simulink model "nlm_1"  (Simulink 5.0)
settings: Solver=ode45  StartTime=0.0  StopTime=600  RelTol=1e-3
libraries: dspsigops x17, fixpt_lib_4 x4
settings Model: Creator=svenhoffmann  LastModifiedBy=svenhoffmann  ExtModeAutoUpdateStatusClock=off  OutputSaveName=yp

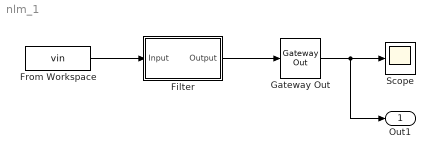
== system nlm_1 ==
  Filter : Subsystem  Tag=FilterWizardSubSystem
  From Workspace : FromWorkspace  VariableName=vin  SampleTime=1
  Gateway Out : fixpt_lib_4/Data Type/Gateway Out  OutRealWorld=Real World Value  OutBuiltInType=double  DoSatur=off
  Scope : Scope
      settings: TimeRange=600  YMin=-0.1  YMax=0.15
  Out1 : Outport
  wires:
  From Workspace/1 -> Filter/1(Input)
  Filter/1(Output) -> Gateway Out/1
  Gateway Out/1 -> Scope/1, Out1/1

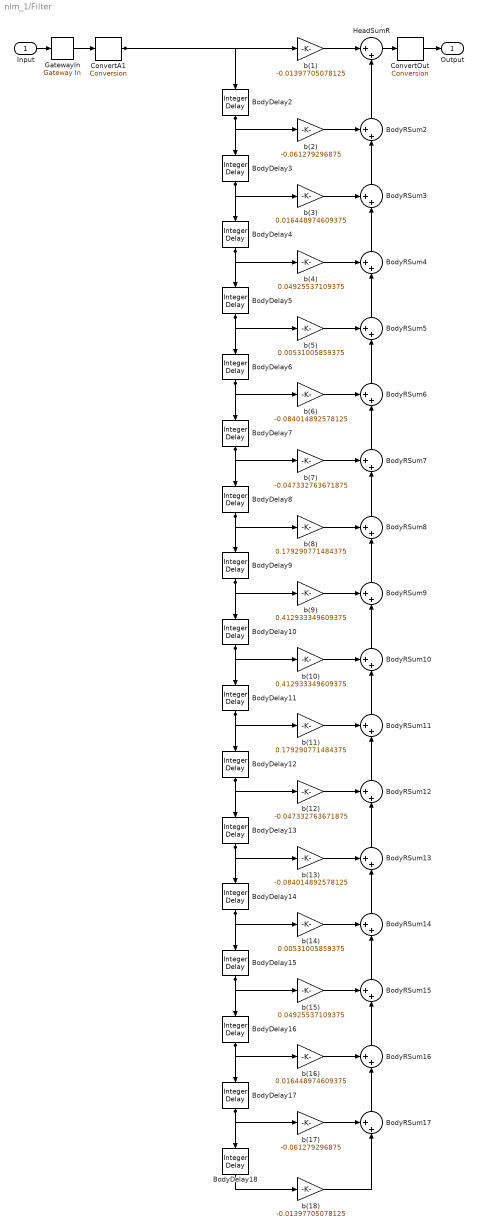
== system nlm_1/Filter ==
  Input : Inport
  BodyDelay{2..18} (17 alike) : dspsigops/Integer Delay  Orientation=down  delay=1  ic=0  reset_popup=None
  BodyRSum{2..17} (16 alike) : Sum  Orientation=up  Inputs=++|  ShowAdditionalParam=on  OutDataTypeMode=Specify via dialog  OutDataType=sfix(32)  OutScaling=2^-30  SaturateOnIntegerOverflow=on  LockScale=on
  ConvertA1 : fixpt_lib_4/Data Type/Conversion  ConvertRealWorld=Real World Value  OutputDataTypeScalingMode=Specify via dialog  OutDataType=sfix(16)  OutScaling=2^-15  DoSatur=on
      settings: LockScale=on
  ConvertOut : fixpt_lib_4/Data Type/Conversion  ConvertRealWorld=Real World Value  OutputDataTypeScalingMode=Specify via dialog  OutDataType=sfix(16)  OutScaling=2^-15  DoSatur=on
      settings: LockScale=on
  GatewayIn : fixpt_lib_4/Data Type/Gateway In  InRealWorld=Real World Value  OutputDataTypeScalingMode=Specify via dialog  OutDataType=sfix(16)  OutScaling=2^-15  DoSatur=on
      settings: LockScale=on
  HeadSumR : Sum  Inputs=|++  ShowAdditionalParam=on  OutDataTypeMode=Specify via dialog  OutDataType=sfix(32)  OutScaling=2^-30  SaturateOnIntegerOverflow=on  LockScale=on
  b(1) : Gain  Gain=-0.01397705078125  ShowAdditionalParam=on  ParameterDataType=float('double')  OutDataTypeMode=Specify via dialog  OutScaling=2^-15  SaturateOnIntegerOverflow=on  LockScale=on
  b(10) : Gain  Gain=0.412933349609375  ShowAdditionalParam=on  ParameterDataType=float('double')  OutDataTypeMode=Specify via dialog  OutScaling=2^-15  SaturateOnIntegerOverflow=on  LockScale=on
  b(11) : Gain  Gain=0.179290771484375  ShowAdditionalParam=on  ParameterDataType=float('double')  OutDataTypeMode=Specify via dialog  OutScaling=2^-15  SaturateOnIntegerOverflow=on  LockScale=on
  b(12) : Gain  Gain=-0.047332763671875  ShowAdditionalParam=on  ParameterDataType=float('double')  OutDataTypeMode=Specify via dialog  OutScaling=2^-15  SaturateOnIntegerOverflow=on  LockScale=on
  b(13) : Gain  Gain=-0.084014892578125  ShowAdditionalParam=on  ParameterDataType=float('double')  OutDataTypeMode=Specify via dialog  OutScaling=2^-15  SaturateOnIntegerOverflow=on  LockScale=on
  b(14) : Gain  Gain=0.00531005859375  ShowAdditionalParam=on  ParameterDataType=float('double')  OutDataTypeMode=Specify via dialog  OutScaling=2^-15  SaturateOnIntegerOverflow=on  LockScale=on
  b(15) : Gain  Gain=0.04925537109375  ShowAdditionalParam=on  ParameterDataType=float('double')  OutDataTypeMode=Specify via dialog  OutScaling=2^-15  SaturateOnIntegerOverflow=on  LockScale=on
  b(16) : Gain  Gain=0.016448974609375  ShowAdditionalParam=on  ParameterDataType=float('double')  OutDataTypeMode=Specify via dialog  OutScaling=2^-15  SaturateOnIntegerOverflow=on  LockScale=on
  b(17) : Gain  Gain=-0.061279296875  ShowAdditionalParam=on  ParameterDataType=float('double')  OutDataTypeMode=Specify via dialog  OutScaling=2^-15  SaturateOnIntegerOverflow=on  LockScale=on
  b(18) : Gain  Gain=-0.01397705078125  ShowAdditionalParam=on  ParameterDataType=float('double')  OutDataTypeMode=Specify via dialog  OutScaling=2^-15  SaturateOnIntegerOverflow=on  LockScale=on
  b(2) : Gain  Gain=-0.061279296875  ShowAdditionalParam=on  ParameterDataType=float('double')  OutDataTypeMode=Specify via dialog  OutScaling=2^-15  SaturateOnIntegerOverflow=on  LockScale=on
  b(3) : Gain  Gain=0.016448974609375  ShowAdditionalParam=on  ParameterDataType=float('double')  OutDataTypeMode=Specify via dialog  OutScaling=2^-15  SaturateOnIntegerOverflow=on  LockScale=on
  b(4) : Gain  Gain=0.04925537109375  ShowAdditionalParam=on  ParameterDataType=float('double')  OutDataTypeMode=Specify via dialog  OutScaling=2^-15  SaturateOnIntegerOverflow=on  LockScale=on
  b(5) : Gain  Gain=0.00531005859375  ShowAdditionalParam=on  ParameterDataType=float('double')  OutDataTypeMode=Specify via dialog  OutScaling=2^-15  SaturateOnIntegerOverflow=on  LockScale=on
  b(6) : Gain  Gain=-0.084014892578125  ShowAdditionalParam=on  ParameterDataType=float('double')  OutDataTypeMode=Specify via dialog  OutScaling=2^-15  SaturateOnIntegerOverflow=on  LockScale=on
  b(7) : Gain  Gain=-0.047332763671875  ShowAdditionalParam=on  ParameterDataType=float('double')  OutDataTypeMode=Specify via dialog  OutScaling=2^-15  SaturateOnIntegerOverflow=on  LockScale=on
  b(8) : Gain  Gain=0.179290771484375  ShowAdditionalParam=on  ParameterDataType=float('double')  OutDataTypeMode=Specify via dialog  OutScaling=2^-15  SaturateOnIntegerOverflow=on  LockScale=on
  b(9) : Gain  Gain=0.412933349609375  ShowAdditionalParam=on  ParameterDataType=float('double')  OutDataTypeMode=Specify via dialog  OutScaling=2^-15  SaturateOnIntegerOverflow=on  LockScale=on
  Output : Outport
  wires:
  GatewayIn/1 -> ConvertA1/1
  Input/1 -> GatewayIn/1
  ConvertOut/1 -> Output/1
  HeadSumR/1 -> ConvertOut/1
  ConvertA1/1 -> b(1)/1, BodyDelay2/1
  b(18)/1 -> BodyRSum17/2
  BodyDelay18/1 -> b(18)/1
  BodyRSum17/1 -> BodyRSum16/2
  b(17)/1 -> BodyRSum17/1
  BodyDelay17/1 -> BodyDelay18/1, b(17)/1
  BodyRSum16/1 -> BodyRSum15/2
  b(16)/1 -> BodyRSum16/1
  BodyDelay16/1 -> BodyDelay17/1, b(16)/1
  BodyRSum15/1 -> BodyRSum14/2
  b(15)/1 -> BodyRSum15/1
  BodyDelay15/1 -> BodyDelay16/1, b(15)/1
  BodyRSum14/1 -> BodyRSum13/2
  b(14)/1 -> BodyRSum14/1
  BodyDelay14/1 -> BodyDelay15/1, b(14)/1
  BodyRSum13/1 -> BodyRSum12/2
  b(13)/1 -> BodyRSum13/1
  BodyDelay13/1 -> BodyDelay14/1, b(13)/1
  BodyRSum12/1 -> BodyRSum11/2
  b(12)/1 -> BodyRSum12/1
  BodyDelay12/1 -> BodyDelay13/1, b(12)/1
  BodyRSum11/1 -> BodyRSum10/2
  b(11)/1 -> BodyRSum11/1
  BodyDelay11/1 -> BodyDelay12/1, b(11)/1
  BodyRSum10/1 -> BodyRSum9/2
  b(10)/1 -> BodyRSum10/1
  BodyDelay10/1 -> BodyDelay11/1, b(10)/1
  BodyRSum9/1 -> BodyRSum8/2
  b(9)/1 -> BodyRSum9/1
  BodyDelay9/1 -> BodyDelay10/1, b(9)/1
  BodyRSum8/1 -> BodyRSum7/2
  b(8)/1 -> BodyRSum8/1
  BodyDelay8/1 -> BodyDelay9/1, b(8)/1
  BodyRSum7/1 -> BodyRSum6/2
  b(7)/1 -> BodyRSum7/1
  BodyDelay7/1 -> BodyDelay8/1, b(7)/1
  BodyRSum6/1 -> BodyRSum5/2
  b(6)/1 -> BodyRSum6/1
  BodyDelay6/1 -> BodyDelay7/1, b(6)/1
  BodyRSum5/1 -> BodyRSum4/2
  b(5)/1 -> BodyRSum5/1
  BodyDelay5/1 -> BodyDelay6/1, b(5)/1
  BodyRSum4/1 -> BodyRSum3/2
  b(4)/1 -> BodyRSum4/1
  BodyDelay4/1 -> BodyDelay5/1, b(4)/1
  BodyRSum3/1 -> BodyRSum2/2
  b(3)/1 -> BodyRSum3/1
  BodyDelay3/1 -> BodyDelay4/1, b(3)/1
  BodyRSum2/1 -> HeadSumR/2
  b(2)/1 -> BodyRSum2/1
  BodyDelay2/1 -> BodyDelay3/1, b(2)/1
  b(1)/1 -> HeadSumR/1
